simulink model "Tutorial_Simulink_3"  (R2024a)
settings: Solver=VariableStepAuto  StartTime=0.0  StopTime=10.0  RelTol=1e-3
settings Model: Creator=gzipprich  LastModifiedBy=gzipprich

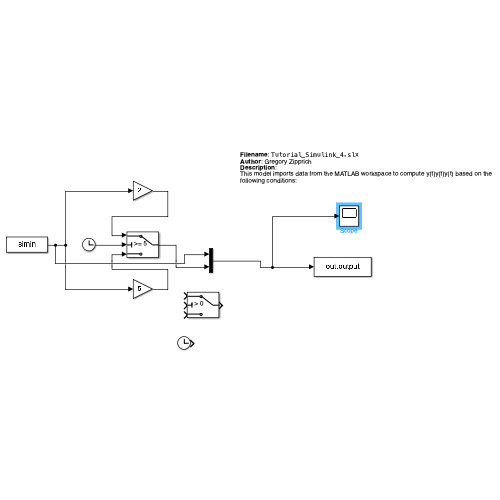
[thumbnail: Simulink's stored preview of the top-level diagram]
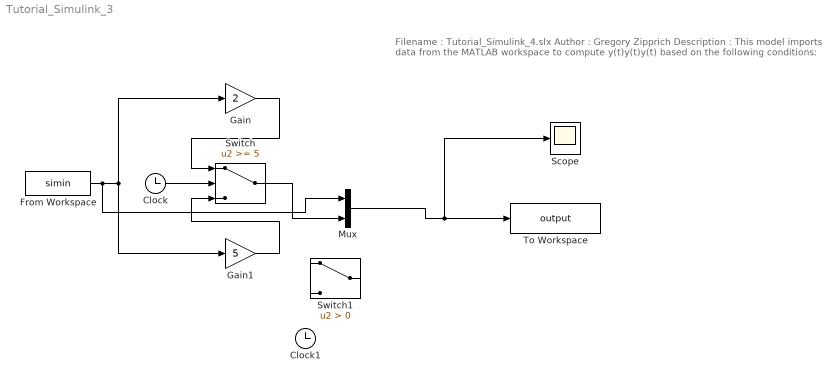
== system Tutorial_Simulink_3 ==
  note: Filename : Tutorial_Simulink_4.slx
      | Author : Gregory Zipprich
      | Description :
      | This model imports data from the MATLAB workspace to compute y(t)y(t)y(t) based on the following conditions:
  Clock : Clock
  Clock1 : Clock
  From Workspace : FromWorkspace  VariableName=simin  SampleTime=.05
  Gain : Gain  Gain=2
  Gain1 : Gain  Gain=5
  Mux : Mux  Inputs=2
  Scope : Scope
  Switch : Switch  Threshold=5  SaturateOnIntegerOverflow=off  InputSameDT=off
  Switch1 : Switch  Criteria=u2 > Threshold  SaturateOnIntegerOverflow=off  InputSameDT=off
  To Workspace : ToWorkspace  VariableName=output  SaveFormat=Timeseries  SampleTime=-1
  wires:
  Clock/1 -> Switch/2
  From Workspace/1 -> Mux/1, Gain/1, Gain1/1
  Mux/1 -> Scope/1, To Workspace/1
  Gain/1 -> Switch/1
  Gain1/1 -> Switch/3
  Switch/1 -> Mux/2
